simulink model "EZQ4sRStEnCtrl"  (R2018b)
settings: Solver=FixedStepDiscrete  StartTime=0.0  StopTime=10.0  FixedStep=0.01  RelTol=1e-3
undefined symbols (not defined in the file or in its folder): data, KeSMSw4SAcsMdSecRwLtStBkReclnRstTm_Val, KeSMSw4SSecRwRtStLgrstOtwdInwdClosePos1_Val, KeSMSw4SSecRwRtStLgrstUpwdDnwdClosePos1_Val, KeSMSw4SSecRwRtStLgrstUpwdDnwdClosePos2_Val, SecRwRtStBkReclnEn_Clear, SecRwRtStBkReclnEn_Set, SecRwRtStFtrstEn_Clear, SecRwRtStFtrstEn_Set, SecRwRtStFwdBkwdEn_Clear, SecRwRtStFwdBkwdEn_Set, SecRwRtStLgrstInwdOtwdEn_Clear, SecRwRtStLgrstInwdOtwdEn_Set, SecRwRtStLgrstUpwdDnwdEn_Clear, SecRwRtStLgrstUpwdDnwdEn_Set
libraries: simulink x1
settings Model: Creator=sn2xws  LastModifiedBy=sn2xws
settings Model: ModifiedHistory=|
  | 2023.8.1 V2.0.0 CR421790 增加模式21-26
  | 2023.10.17
  | V2.3.0 Bug 554442 4座2L便利下车，乘员离开座椅后，靠背位置没有从17%运动到50%
  | 在empty后面增加一个延时
settings DataIOCC: SaveFormat=StructureWithTime
settings OptimizationCC: DefaultParameterBehavior=Inlined  EnhancedBackFolding=on  PassReuseOutputArgsAs=Individual arguments  ZeroExternalMemoryAtStartup=off  ZeroInternalMemoryAtStartup=off  OptimizeBlockOrder=speed  DifferentSizesBufferReuse=on  OptimizationCustomize=off
settings DebuggingCC: ParameterTunabilityLossMsg=error
settings SFSimCC: MATLABDynamicMemAlloc=off
settings RTWCC: SystemTargetFile=autosar.tlc  GenCodeOnly=on  TemplateMakefile=ert_default_tmf  Description=AUTOSAR  GenerateReport=on  IncludeHyperlinkInReport=on  LaunchReport=on  GenerateTraceInfo=on  GenerateTraceReport=on  GenerateTraceReportSl=on  GenerateTraceReportSf=on  GenerateTraceReportEml=on  GenerateCodeMetricsReport=on
settings CodeAppCC: ForceParamTrailComments=on  IgnoreCustomStorageClasses=off  OperatorAnnotations=on  SimulinkDataObjDesc=on  SFDataObjDesc=on  InsertBlockDesc=on
settings STFCustomTargetCC: TargetLangStandard=C99 (ISO)  MultiwordLength=256  ParMdlRefBuildCompliant=on  CompOptLevelCompliant=on  IncludeMdlTerminateFcn=off  CombineOutputUpdateFcns=on  SuppressErrorStatus=on  ERTCustomFileBanners=on  SupportNonFinite=off  SupportComplex=off  SupportContinuousTime=off  SupportNonInlinedSFcns=off  RemoveResetFunc=on  MATLABClassNameForMDSCustomization=Simulink.SoftwareTarget.ERTCustomization  AutosarCompliant=on  UseToolchainInfoCompliant=on  LookupTableObjectStructAxisOrder=2,1,3,4,...  LUTObjectStructOrderEvenSpacing=Size,Table,Breakpoints  SystemTargetFile=autosar.tlc
settings ERTTargetCC: TargetLangStandard=C99 (ISO)  ConcurrentExecutionCompliant=off  IncludeMdlTerminateFcn=off  SuppressErrorStatus=on  SupportNonFinite=off  SupportComplex=off  ModelStepFunctionPrototypeControlCompliant=off  CPPClassGenCompliant=off  AutosarCompliant=on  LookupTableObjectStructAxisOrder=2,1,3,4,...  LUTObjectStructOrderEvenSpacing=Size,Table,Breakpoints  InlinedParameterPlacement=NonHierarchical  ERTCustomFileTemplate=example_file_process.tlc  ERTFilePackagingFormat=Compact

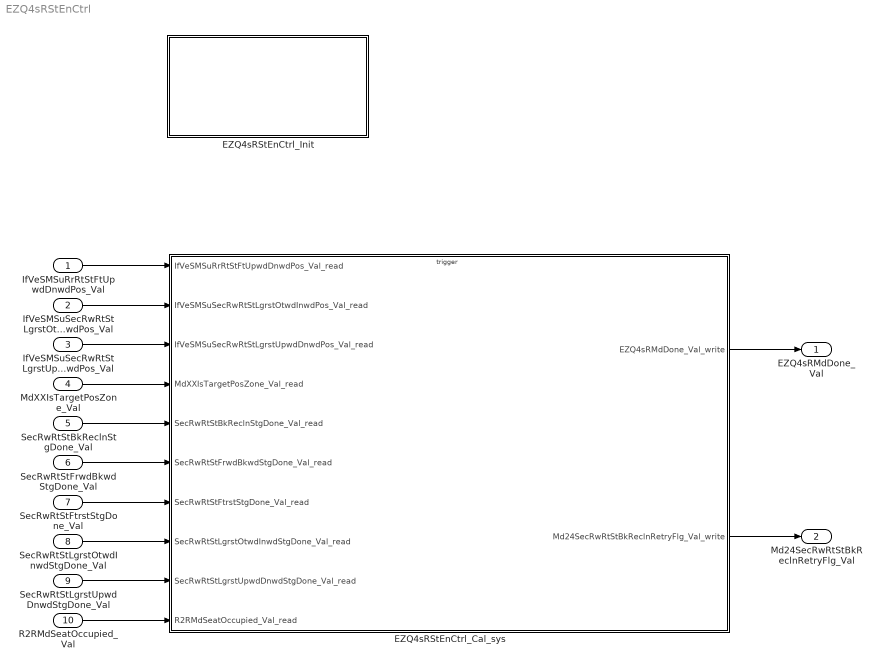
== system EZQ4sRStEnCtrl ==
  IfVeSMSuRrRtStFtUpwdDnwdPos_Val : Inport  OutDataTypeStr=uint16  PortDimensions=1
  IfVeSMSuSecRwRtStLgrstOtwdInwdPos_Val : Inport  Port=2  OutDataTypeStr=uint16  PortDimensions=1
  IfVeSMSuSecRwRtStLgrstUpwdDnwdPos_Val : Inport  Port=3  OutDataTypeStr=uint16  PortDimensions=1
  MdXXIsTargetPosZone_Val : Inport  Port=4  OutDataTypeStr=uint32  PortDimensions=1
  SecRwRtStBkReclnStgDone_Val : Inport  Port=5  OutDataTypeStr=boolean  PortDimensions=1
  SecRwRtStFrwdBkwdStgDone_Val : Inport  Port=6  OutDataTypeStr=boolean  PortDimensions=1
  SecRwRtStFtrstStgDone_Val : Inport  Port=7  OutDataTypeStr=boolean  PortDimensions=1
  SecRwRtStLgrstOtwdInwdStgDone_Val : Inport  Port=8  OutDataTypeStr=boolean  PortDimensions=1
  SecRwRtStLgrstUpwdDnwdStgDone_Val : Inport  Port=9  OutDataTypeStr=boolean  PortDimensions=1
  R2RMdSeatOccupied_Val : Inport  Port=10  OutDataTypeStr=boolean  PortDimensions=1
  EZQ4sRStEnCtrl_Cal_sys : Subsystem
  EZQ4sRStEnCtrl_Init : Subsystem
  EZQ4sRMdDone_Val : Outport  OutDataTypeStr=uint8  PortDimensions=1
  Md24SecRwRtStBkReclnRetryFlg_Val : Outport  Port=2  OutDataTypeStr=boolean  PortDimensions=1
  wires:
  IfVeSMSuRrRtStFtUpwdDnwdPos_Val/1 -> EZQ4sRStEnCtrl_Cal_sys/1(IfVeSMSuRrRtStFtUpwdDnwdPos_Val_read)
  IfVeSMSuSecRwRtStLgrstOtwdInwdPos_Val/1 -> EZQ4sRStEnCtrl_Cal_sys/2(IfVeSMSuSecRwRtStLgrstOtwdInwdPos_Val_read)
  IfVeSMSuSecRwRtStLgrstUpwdDnwdPos_Val/1 -> EZQ4sRStEnCtrl_Cal_sys/3(IfVeSMSuSecRwRtStLgrstUpwdDnwdPos_Val_read)
  MdXXIsTargetPosZone_Val/1 -> EZQ4sRStEnCtrl_Cal_sys/4(MdXXIsTargetPosZone_Val_read)
  SecRwRtStBkReclnStgDone_Val/1 -> EZQ4sRStEnCtrl_Cal_sys/5(SecRwRtStBkReclnStgDone_Val_read)
  SecRwRtStFrwdBkwdStgDone_Val/1 -> EZQ4sRStEnCtrl_Cal_sys/6(SecRwRtStFrwdBkwdStgDone_Val_read)
  SecRwRtStFtrstStgDone_Val/1 -> EZQ4sRStEnCtrl_Cal_sys/7(SecRwRtStFtrstStgDone_Val_read)
  SecRwRtStLgrstOtwdInwdStgDone_Val/1 -> EZQ4sRStEnCtrl_Cal_sys/8(SecRwRtStLgrstOtwdInwdStgDone_Val_read)
  SecRwRtStLgrstUpwdDnwdStgDone_Val/1 -> EZQ4sRStEnCtrl_Cal_sys/9(SecRwRtStLgrstUpwdDnwdStgDone_Val_read)
  EZQ4sRStEnCtrl_Cal_sys/1(EZQ4sRMdDone_Val_write) -> EZQ4sRMdDone_Val/1
  R2RMdSeatOccupied_Val/1 -> EZQ4sRStEnCtrl_Cal_sys/10(R2RMdSeatOccupied_Val_read)
  EZQ4sRStEnCtrl_Cal_sys/2(Md24SecRwRtStBkReclnRetryFlg_Val_write) -> Md24SecRwRtStBkReclnRetryFlg_Val/1

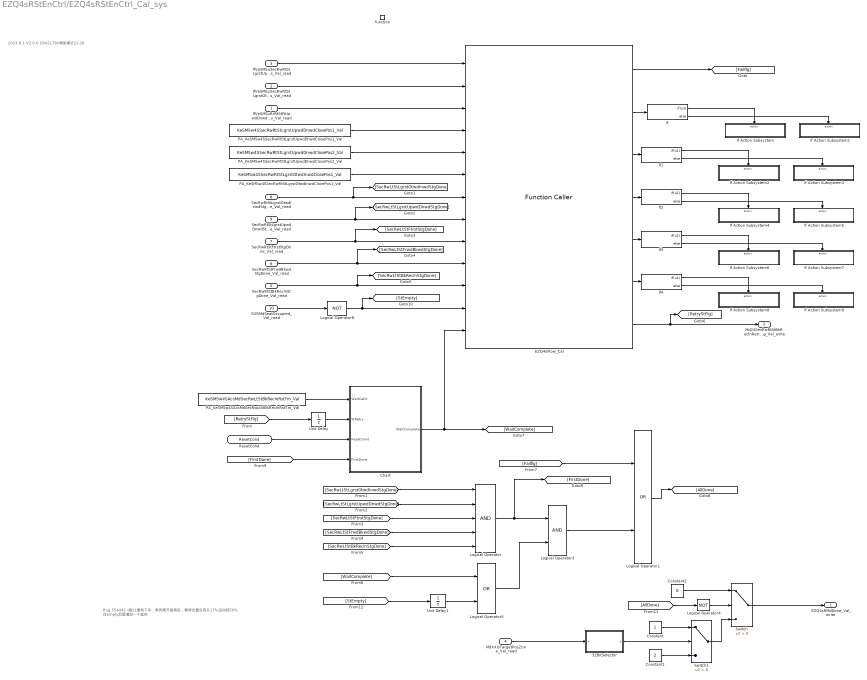
== system EZQ4sRStEnCtrl/EZQ4sRStEnCtrl_Cal_sys ==
  note: Bug 554442 4座2L便利下车，乘员离开座椅后，靠背位置没有从17%运动到50%
      | 在empty后面增加一个延时
  note: 2023.8.1 V2.0.0 CR421790 增加模式21-26
  IfVeSMSuRrRtStFtUpwdDnwdPos_Val_read : Inport
  IfVeSMSuSecRwRtStLgrstOtwdInwdPos_Val_read : Inport  Port=2
  IfVeSMSuSecRwRtStLgrstUpwdDnwdPos_Val_read : Inport  Port=3
  MdXXIsTargetPosZone_Val_read : Inport  Port=4
  SecRwRtStBkReclnStgDone_Val_read : Inport  Port=5
  SecRwRtStFrwdBkwdStgDone_Val_read : Inport  Port=6
  SecRwRtStFtrstStgDone_Val_read : Inport  Port=7
  SecRwRtStLgrstOtwdInwdStgDone_Val_read : Inport  Port=8
  SecRwRtStLgrstUpwdDnwdStgDone_Val_read : Inport  Port=9
  R2RMdSeatOccupied_Val_read : Inport  Port=10
  function : TriggerPort  TriggerType=function-call  IsSimulinkFunction=on  FunctionName=EZQ4sRStEnCtrl_Cal  VariantControl=(inherit)
  32BitSelector : Subsystem  mask(32 Bit Selector){BitNum=23}
      mask prompts: BitNum "Select Bit Number"
      mask help: Allows selection of a particular bit (0-31) out of a packed word up to 32 bits long. Output will be true if the bit number selected via the mask parameter is equal to one.
      mask TypeOptions BitNum: 0 | 1 | 2 | 3 | 4 | 5 | 6 | 7 | 8 | 9 | 10 | 11 | 12 | 13 | 14 | 15 | 16 | 17 | 18 | 19 | 20 | 21 | 22 | 23 | 24 | 25 | 26 | 27 | 28 | 29 | 30 | 31
      mask Display:
      | text(0.5, 0.8,'BIT','horizontalAlignment','center')
      | text(0.5, 0.5,'SELECTOR','horizontalAlignment','center')
      | text(0.5, 0.2,['-- Bit ',char(get_param(gcb,'BitNum')),' --'],'horizontalAlignment','center')
  Chart : Stateflow chart  TreatAsAtomicUnit=on
  Constant : Constant  OutDataTypeStr=uint8
  Constant1 : Constant  Value=2  OutDataTypeStr=uint8
  Constant2 : Constant  Value=0  OutDataTypeStr=uint8
  EZQ4sFlow_Cal : FunctionCaller  FunctionPrototype=[Failflg,LgrstInwdOtwdEn,LgrstUpwdDnwdEn,FtrstEn,FrwdBkwdEn,BkReclnEn,RetryStFlg] = EZQ4sFlow_Cal(LgrstUpwdDnwdPos,LgrstOtwdInwdPos,FtUpwdDnwdPos,CloseDnwdPos1,CloseDnwdPos2,CloseOtwdPos1,LgrstInwdStgDone,LgrstUpwdStgDone,FtrstStgDone,FrwdBkwdStgDone,BkReclnStgDone,StEmpty,WaitComplete)  InputArgumentSpecifications=uint16(1), uint16(1), uint16(1), uint16(1), uint16(1), uint16(1), boolean(true), boolean(true), boolean(true), boolean(true), boolean(true), boolean(true), boolean(true)  OutputArgumentSpecifications=boolean(true), boolean(true), boolean(true), boolean(true), boolean(true), boolean(true), boolean(true)
  If{,1..4} (5 alike) : If  IfExpression=u1
  If Action Subsystem : Subsystem  TreatAsAtomicUnit=on
  If Action Subsystem1 : Subsystem  TreatAsAtomicUnit=on
  If Action Subsystem2 : Subsystem  TreatAsAtomicUnit=on
  If Action Subsystem3 : Subsystem  TreatAsAtomicUnit=on
  If Action Subsystem4 : Subsystem  TreatAsAtomicUnit=on
  If Action Subsystem5 : Subsystem  TreatAsAtomicUnit=on
  If Action Subsystem6 : Subsystem  TreatAsAtomicUnit=on
  If Action Subsystem7 : Subsystem  TreatAsAtomicUnit=on
  If Action Subsystem8 : Subsystem  TreatAsAtomicUnit=on
  If Action Subsystem9 : Subsystem  TreatAsAtomicUnit=on
  Logical Operator : Logic  Inputs=5  AllPortsSameDT=off  OutDataTypeStr=boolean
  Logical Operator1 : Logic  Operator=OR  AllPortsSameDT=off  OutDataTypeStr=boolean
  Logical Operator3 : Logic  AllPortsSameDT=off  OutDataTypeStr=boolean
  Logical Operator4 : Logic  Operator=NOT  AllPortsSameDT=off  OutDataTypeStr=boolean
  Logical Operator5 : Logic  Operator=OR  AllPortsSameDT=off  OutDataTypeStr=boolean
  Logical Operator8 : Logic  Operator=NOT  AllPortsSameDT=off  OutDataTypeStr=boolean
  PA_KeSMSw4SAcsMdSecRwLtStBkReclnRstTm_Val : Constant  Value=KeSMSw4SAcsMdSecRwLtStBkReclnRstTm_Val
  PA_KeSMSw4SSecRwRtStLgrstOtwdInwdClosePos1_Val : Constant  Value=KeSMSw4SSecRwRtStLgrstOtwdInwdClosePos1_Val
  PA_KeSMSw4SSecRwRtStLgrstUpwdDnwdClosePos1_Val : Constant  Value=KeSMSw4SSecRwRtStLgrstUpwdDnwdClosePos1_Val
  PA_KeSMSw4SSecRwRtStLgrstUpwdDnwdClosePos2_Val : Constant  Value=KeSMSw4SSecRwRtStLgrstUpwdDnwdClosePos2_Val
  Switch : Switch  Criteria=u2 > Threshold
  Switch1 : Switch  Criteria=u2 > Threshold
  Unit Delay : UnitDelay  SampleTime=-1
  Unit Delay1 : UnitDelay  SampleTime=-1
  ResetCond : ArgIn  OutDataTypeStr=boolean  ArgumentName=ResetCond
  EZQ4sRMdDone_Val_write : Outport
      settings: EnsureOutportIsVirtual=on
  Md24SecRwRtStBkReclnRetryFlg_Val_write : Outport  Port=2
      settings: EnsureOutportIsVirtual=on
  wires:
  IfVeSMSuSecRwRtStLgrstUpwdDnwdPos_Val_read/1 -> EZQ4sFlow_Cal/1
  IfVeSMSuSecRwRtStLgrstOtwdInwdPos_Val_read/1 -> EZQ4sFlow_Cal/2
  IfVeSMSuRrRtStFtUpwdDnwdPos_Val_read/1 -> EZQ4sFlow_Cal/3
  PA_KeSMSw4SSecRwRtStLgrstUpwdDnwdClosePos1_Val/1 -> EZQ4sFlow_Cal/4
  PA_KeSMSw4SSecRwRtStLgrstUpwdDnwdClosePos2_Val/1 -> EZQ4sFlow_Cal/5
  PA_KeSMSw4SSecRwRtStLgrstOtwdInwdClosePos1_Val/1 -> EZQ4sFlow_Cal/6
  SecRwRtStLgrstOtwdInwdStgDone_Val_read/1 -> [SecRwLtStLgrstOtwdInwdStgDone], EZQ4sFlow_Cal/7
  SecRwRtStLgrstUpwdDnwdStgDone_Val_read/1 -> [SecRwLtStLgrstUpwdDnwdStgDone], EZQ4sFlow_Cal/8
  SecRwRtStFtrstStgDone_Val_read/1 -> [SecRwLtStFtrstStgDone], EZQ4sFlow_Cal/9
  SecRwRtStFrwdBkwdStgDone_Val_read/1 -> [SecRwLtStFrwdBkwdStgDone], EZQ4sFlow_Cal/10
  SecRwRtStBkReclnStgDone_Val_read/1 -> [SecRwLtStBkReclnStgDone], EZQ4sFlow_Cal/11
  Unit Delay/1 -> Chart/2(StRetry)
  ResetCond/1 -> Chart/3(ResetCond)
  [RetryStFlg] -> Unit Delay/1
  PA_KeSMSw4SAcsMdSecRwLtStBkReclnRstTm_Val/1 -> Chart/1(WaitCalib)
  [SecRwLtStLgrstUpwdDnwdStgDone] -> Logical Operator/2
  [SecRwLtStLgrstOtwdInwdStgDone] -> Logical Operator/1
  [SecRwLtStFtrstStgDone] -> Logical Operator/3
  32BitSelector/1(y) -> Switch1/2
  Switch/1 -> EZQ4sRMdDone_Val_write/1
  [SecRwLtStBkReclnStgDone] -> Logical Operator/5
  Chart/1(WaitComplete) -> EZQ4sFlow_Cal/13, [WaitComplete]
  [WaitComplete] -> Logical Operator5/1
  Logical Operator1/1 -> [AllDone]
  MdXXIsTargetPosZone_Val_read/1 -> 32BitSelector/1(x)
  [Failflg] -> Logical Operator1/1
  [SecRwLtStFrwdBkwdStgDone] -> Logical Operator/4
  Switch1/1 -> Switch/3
  EZQ4sFlow_Cal/1 -> [Failflg]
  EZQ4sFlow_Cal/7 -> Md24SecRwRtStBkReclnRetryFlg_Val_write/1, [RetryStFlg]
  R2RMdSeatOccupied_Val_read/1 -> Logical Operator8/1
  If/1 -> If Action Subsystem/Action
  If/2 -> If Action Subsystem1/Action
  EZQ4sFlow_Cal/2 -> If/1
  If1/2 -> If Action Subsystem3/Action
  If1/1 -> If Action Subsystem2/Action
  EZQ4sFlow_Cal/3 -> If1/1
  If2/1 -> If Action Subsystem4/Action
  If2/2 -> If Action Subsystem5/Action
  EZQ4sFlow_Cal/4 -> If2/1
  If3/2 -> If Action Subsystem7/Action
  If3/1 -> If Action Subsystem6/Action
  EZQ4sFlow_Cal/5 -> If3/1
  If4/1 -> If Action Subsystem8/Action
  If4/2 -> If Action Subsystem9/Action
  EZQ4sFlow_Cal/6 -> If4/1
  [FirstDone] -> Chart/4(FirstDone)
  Logical Operator3/1 -> Logical Operator1/2
  Logical Operator/1 -> [FirstDone], Logical Operator3/1
  Logical Operator5/1 -> Logical Operator3/2
  Logical Operator8/1 -> [StEmpty], EZQ4sFlow_Cal/12
  [StEmpty] -> Unit Delay1/1
  [AllDone] -> Logical Operator4/1
  Constant2/1 -> Switch/1
  Constant/1 -> Switch1/1
  Constant1/1 -> Switch1/3
  Logical Operator4/1 -> Switch/2
  Unit Delay1/1 -> Logical Operator5/2

== system EZQ4sRStEnCtrl/EZQ4sRStEnCtrl_Init ==
  Event Listener : EventListener  EventName=reset

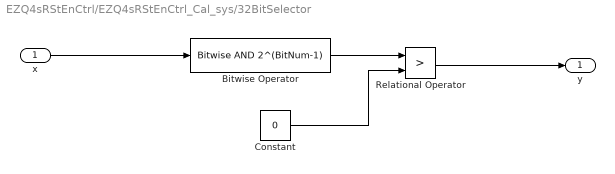
== system EZQ4sRStEnCtrl/EZQ4sRStEnCtrl_Cal_sys/32BitSelector ==
  x : Inport
  Bitwise Operator : simulink/Logic and Bit Operations/Bitwise Operator  logicop=AND  UseBitMask=on  BitMask=2^(BitNum-1)  BitMaskRealWorld=Stored Integer
  Constant : Constant  Value=0  OutDataTypeStr=uint32
  Relational Operator : RelationalOperator  Operator=>  OutDataTypeStr=boolean  RndMeth=Simplest
  y : Outport
  wires:
  Relational Operator/1 -> y/1
  Constant/1 -> Relational Operator/2
  x/1 -> Bitwise Operator/1
  Bitwise Operator/1 -> Relational Operator/1

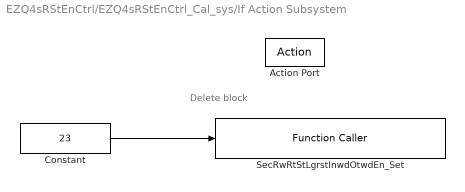
== system EZQ4sRStEnCtrl/EZQ4sRStEnCtrl_Cal_sys/If Action Subsystem ==
  note: Delete block
  Action Port : ActionPort  ActionType=then
  Constant : Constant  Value=23  OutDataTypeStr=uint8
  SecRwRtStLgrstInwdOtwdEn_Set : FunctionCaller  FunctionPrototype=SecRwRtStLgrstInwdOtwdEn_Set(data)  InputArgumentSpecifications=uint8(1)
  wires:
  Constant/1 -> SecRwRtStLgrstInwdOtwdEn_Set/1

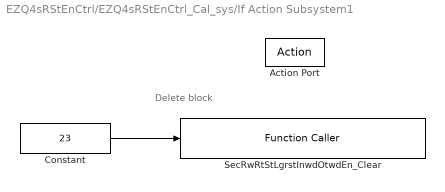
== system EZQ4sRStEnCtrl/EZQ4sRStEnCtrl_Cal_sys/If Action Subsystem1 ==
  note: Delete block
  Action Port : ActionPort  ActionType=else
  Constant : Constant  Value=23  OutDataTypeStr=uint8
  SecRwRtStLgrstInwdOtwdEn_Clear : FunctionCaller  FunctionPrototype=SecRwRtStLgrstInwdOtwdEn_Clear(data)  InputArgumentSpecifications=uint8(1)
  wires:
  Constant/1 -> SecRwRtStLgrstInwdOtwdEn_Clear/1

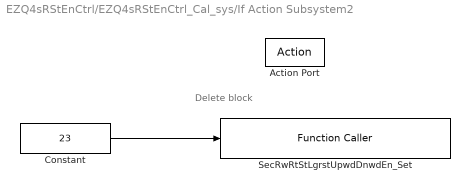
== system EZQ4sRStEnCtrl/EZQ4sRStEnCtrl_Cal_sys/If Action Subsystem2 ==
  note: Delete block
  Action Port : ActionPort  ActionType=then
  Constant : Constant  Value=23  OutDataTypeStr=uint8
  SecRwRtStLgrstUpwdDnwdEn_Set : FunctionCaller  FunctionPrototype=SecRwRtStLgrstUpwdDnwdEn_Set(data)  InputArgumentSpecifications=uint8(1)
  wires:
  Constant/1 -> SecRwRtStLgrstUpwdDnwdEn_Set/1

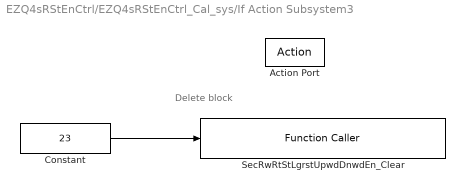
== system EZQ4sRStEnCtrl/EZQ4sRStEnCtrl_Cal_sys/If Action Subsystem3 ==
  note: Delete block
  Action Port : ActionPort  ActionType=else
  Constant : Constant  Value=23  OutDataTypeStr=uint8
  SecRwRtStLgrstUpwdDnwdEn_Clear : FunctionCaller  FunctionPrototype=SecRwRtStLgrstUpwdDnwdEn_Clear(data)  InputArgumentSpecifications=uint8(1)
  wires:
  Constant/1 -> SecRwRtStLgrstUpwdDnwdEn_Clear/1

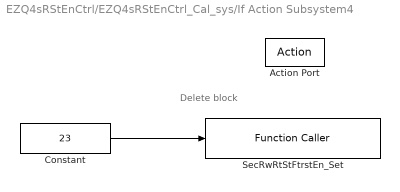
== system EZQ4sRStEnCtrl/EZQ4sRStEnCtrl_Cal_sys/If Action Subsystem4 ==
  note: Delete block
  Action Port : ActionPort  ActionType=then
  Constant : Constant  Value=23  OutDataTypeStr=uint8
  SecRwRtStFtrstEn_Set : FunctionCaller  FunctionPrototype=SecRwRtStFtrstEn_Set(data)  InputArgumentSpecifications=uint8(1)
  wires:
  Constant/1 -> SecRwRtStFtrstEn_Set/1

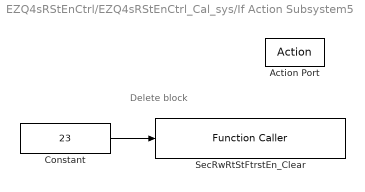
== system EZQ4sRStEnCtrl/EZQ4sRStEnCtrl_Cal_sys/If Action Subsystem5 ==
  note: Delete block
  Action Port : ActionPort  ActionType=else
  Constant : Constant  Value=23  OutDataTypeStr=uint8
  SecRwRtStFtrstEn_Clear : FunctionCaller  FunctionPrototype=SecRwRtStFtrstEn_Clear(data)  InputArgumentSpecifications=uint8(1)
  wires:
  Constant/1 -> SecRwRtStFtrstEn_Clear/1

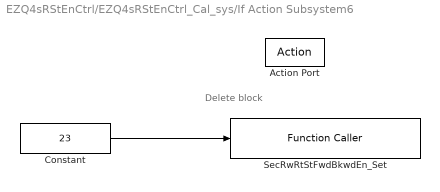
== system EZQ4sRStEnCtrl/EZQ4sRStEnCtrl_Cal_sys/If Action Subsystem6 ==
  note: Delete block
  Action Port : ActionPort  ActionType=then
  Constant : Constant  Value=23  OutDataTypeStr=uint8
  SecRwRtStFwdBkwdEn_Set : FunctionCaller  FunctionPrototype=SecRwRtStFwdBkwdEn_Set(data)  InputArgumentSpecifications=uint8(1)
  wires:
  Constant/1 -> SecRwRtStFwdBkwdEn_Set/1

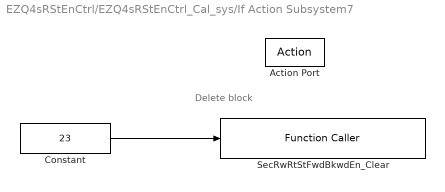
== system EZQ4sRStEnCtrl/EZQ4sRStEnCtrl_Cal_sys/If Action Subsystem7 ==
  note: Delete block
  Action Port : ActionPort  ActionType=else
  Constant : Constant  Value=23  OutDataTypeStr=uint8
  SecRwRtStFwdBkwdEn_Clear : FunctionCaller  FunctionPrototype=SecRwRtStFwdBkwdEn_Clear(data)  InputArgumentSpecifications=uint8(1)
  wires:
  Constant/1 -> SecRwRtStFwdBkwdEn_Clear/1

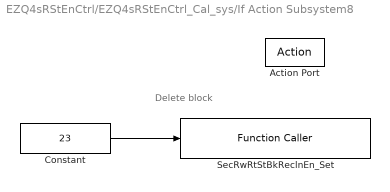
== system EZQ4sRStEnCtrl/EZQ4sRStEnCtrl_Cal_sys/If Action Subsystem8 ==
  note: Delete block
  Action Port : ActionPort  ActionType=then
  Constant : Constant  Value=23  OutDataTypeStr=uint8
  SecRwRtStBkReclnEn_Set : FunctionCaller  FunctionPrototype=SecRwRtStBkReclnEn_Set(data)  InputArgumentSpecifications=uint8(1)
  wires:
  Constant/1 -> SecRwRtStBkReclnEn_Set/1

== system EZQ4sRStEnCtrl/EZQ4sRStEnCtrl_Cal_sys/If Action Subsystem9 ==
  note: Delete block
  Action Port : ActionPort  ActionType=else
  Constant : Constant  Value=23  OutDataTypeStr=uint8
  SecRwRtStBkReclnEn_Clear : FunctionCaller  FunctionPrototype=SecRwRtStBkReclnEn_Clear(data)  InputArgumentSpecifications=uint8(1)
  wires:
  Constant/1 -> SecRwRtStBkReclnEn_Clear/1

== stateflow chart EZQ4sRStEnCtrl/EZQ4sRStEnCtrl_Cal_sys/Chart ==
  (default) -> (junction 16)
  (junction 16) -> (junction 18) [order 1] : [ResetCond]
  (junction 16) -> (junction 21) [order 2]
  (junction 18) -> (junction 23) : {
      | WaitCnt = 0;
      | WaitComplete=false;
      | }
  (junction 23) -> (junction 21)
  (junction 21) -> (junction 26)
  (junction 26) -> (junction 28) [order 1] : [FirstDone]
  (junction 26) -> (junction 30) [order 2]
  (junction 28) -> (junction 32) : {WaitCnt = WaitCnt +1;}
  (junction 32) -> (junction 30)
  (junction 30) -> (junction 5)
  (junction 5) -> (junction 7) [order 1] : [StRetry||WaitCnt>WaitCalib]
  (junction 5) -> (junction 11) [order 2]
  (junction 7) -> (junction 9) : {WaitComplete=true;}
  (junction 9) -> (junction 11)
  (junction 11) -> (junction 14)
  data: WaitCnt local uint16 size=1; WaitCalib input size=1; WaitComplete output boolean size=1; StRetry input size=1; ResetCond input size=1; FirstDone input size=1
